simulink model "wamjc7"  (Simulink 8.3)
settings: Solver=ode4  SolverMode=SingleTasking  StartTime=0.0  StopTime=inf  FixedStep=sample_time  RelTol=1e-3
undefined symbols (not defined in the file): arm_home, arm_home_norest, arm_j2mt, arm_m2jp, b, bit, C, CAN_init, enc_per_rev, FT_init, hand_on, MT_init, puck_I_per_Nm, rotFT2Hand, sample_time, Standard, VL1_init, VL2_init
libraries: xpclib x43, simulink x27, xpcutilitieslib x6, dspmathops x1, dspadpt3 x1, dspindex x1, dspbuff3 x1
(part 2 of 5)

== system wamjc7/Get Arm State/Get FT/Get Force Torque/Recieve and Unpack  Forces and Torques ==
  CAN bit-unpacking 1 : xpclib/CAN/Utilities/CAN bit-unpacking   bitpatterns={[0:15],[16:31],[32:47]}  dtypes={'int32','int32','int32'}
  CAN bit-unpacking 2 : xpclib/CAN/Utilities/CAN bit-unpacking   bitpatterns={[0:15],[16:31],[32:47]}  dtypes={'int32','int32','int32'}
  DocBlock : simulink/Model-Wide Utilities/DocBlock  DocumentType=Text
  ForceToDouble : DataTypeConversion  OutDataTypeStr=double
  Mux1 : Mux  Inputs=3
  Mux2 : Mux  Inputs=3
  "Receive position " : xpclib/CAN/Softing/CAN-AC2-PCI SJA 1000/Receive   board=1  canPort=CAN 1  range=Standard (11-bit)  ids=[bin2dec('10100001010'),bin2dec('10100001011')]  lengths=0  output=Data  inten=on  ts=sample_time  ididx=[8,9]
  TorqueToDouble : DataTypeConversion  OutDataTypeStr=double
  F : Outport
  Tau : Outport  Port=2
  wires:
  "Receive position "/1 -> CAN bit-unpacking 2/1
  "Receive position "/2 -> CAN bit-unpacking 1/1
  Mux1/1 -> TorqueToDouble/1
  CAN bit-unpacking 1/1 -> Mux1/1
  CAN bit-unpacking 1/2 -> Mux1/2
  CAN bit-unpacking 1/3 -> Mux1/3
  TorqueToDouble/1 -> Tau/1
  ForceToDouble/1 -> F/1
  CAN bit-unpacking 2/1 -> Mux2/1
  CAN bit-unpacking 2/2 -> Mux2/2
  CAN bit-unpacking 2/3 -> Mux2/3
  Mux2/1 -> ForceToDouble/1

== system wamjc7/Get Arm State/Get FT/Get Force Torque/Send Get FT ==
  Bit Packing : xpcutilitieslib/Bit Packing   MaskBitPatterns={[0:7]}  MaskPackDataType=double  MaskPackDataSize=[1]
  Send to FTsensor : xpclib/CAN/Softing/CAN-AC2-PCI SJA 1000/Send   board=1  canPort=CAN 1  range=Standard (11-bit)  ids=bin2dec('00000001000')  sizes=[1]  output=off  ts=sample_time  ididx=[0]
  get FT : Constant  Value=[54]  OutDataTypeStr=int8
  wires:
  get FT/1 -> Bit Packing/1
  Bit Packing/1 -> Send to FTsensor/1

== system wamjc7/Subsystem/Plan Arm Trajectory/Send Execution Result/Enabled Subsystem ==
  ExectuionResult : Inport
  Enable : EnablePort
  Pack : xpclib/UDP/Pack  datatypes={'double'}  byteAlign=1
  Send : xpclib/UDP/Send  ipAddress=192.168.1.11  ipPort=3334  localPort=-1  vblLen=off  sampletime=sample_time
  wires:
  ExectuionResult/1 -> Pack/1
  Pack/1 -> Send/1

== matlab function Subsystem/Compute Arm Torque/Dynamics Compensation ==
  data: hand_on input double; tau output double; q input double; qd input double; qdd input double; FTsensor output double
function [tau, FTsensor] = dynamicsComp(hand_on,q,qd,qdd)
%-------------------------------------------------------------------------------------
%   SETUP THE ARM
%-------------------------------------------------------------------------------------    
    DH_a = [0 0 0.045 -0.045 0 0 0];
    DH_d = [0 0 .55 0 0.3 0 0.061];
    DH_alpha = [-pi/2 pi/2 -pi/2 pi/2 -pi/2 pi/2 0];

    m = [8.3936 4.8487 1.7251 2.17266212 0.35655692 0.40915886 0.07548270];
    
    com = zeros(3,7);
    com(:,1) = [0.3506e-3, 132.6795e-3, 0.6286e-3];
    com(:,2) = [-0.2230e-3, -21.3924e-3, 13.3754e-3];
    com(:,3) = [-38.7565e-3, 217.9078e-3, 0.0252e-3];
    com(:,4) = [0.00553408,0.00006822,0.11927695];
    com(:,5) = [0.00005483,0.02886286,0.00148493];
    com(:,6) = [-0.00005923,-0.01686123,0.02419052];
    com(:,7) = [ 0.00014836,0.00007252,-0.00335185];
    
    % Need Inertia matricies
    I = zeros(3,3,7);
    I(:,:,1) = [ 95157.4294e-6,   246.1404e-6,   -95.0183e-6 ;
                   246.1404e-6, 92032.3524e-6,  -962.6725e-6 ;
                   -95.0183e-6,  -962.6725e-6, 59290.5997e-6 ];
    I(:,:,2) = [ 29326.8098e-6,   -43.3994e-6,  -129.2942e-6 ;
                   -43.3994e-6, 20781.5826e-6,  1348.6924e-6 ;
                  -129.2942e-6,  1348.6924e-6, 22807.3271e-6 ];
    I(:,:,3) = [ 56662.2970e-6, -2321.6892e-6,     8.2125e-6 ;
                 -2321.6892e-6,  3158.0509e-6,   -16.6307e-6 ;
                     8.2125e-6,   -16.6307e-6, 56806.6024e-6 ];
    I(:,:,4) = [  0.01067491,  0.00004503, -0.00135557 ;
                  0.00004503,  0.01058659, -0.00011002 ;
                 -0.00135557, -0.00011002,  0.00282036 ];
    I(:,:,5) = [  0.00037112, -0.00000008, -0.00000003 ;
                 -0.00000008,  0.00019434, -0.00001613 ;
                 -0.00000003, -0.00001613,  0.00038209 ];
    I(:,:,6) =  [  0.00054889,  0.00000019, -0.00000010 ;
                   0.00000019,  0.00023846, -0.00004430 ;
                  -0.00000010, -0.00004430,  0.00045133 ];
    I(:,:,7) = [ 0.00003911, 0.00000019, 0.00000000 ;      % WAM without hand
                 0.00000019, 0.00003877, 0.00000000 ;
                 0.00000000, 0.00000000, 0.00007614 ];
    
    %Link Gear Ratio
    % The differential drive mechanism was ignored here because it's not
    % supported by the robotic toolbox yet.
    % Please refer to: http://www.me.unm.edu/~starr/research/WAM_MassParams_AA-00.pdf
    G = zeros(7,1);
    G(1) =  42.00;
    G(2) =  28.25;
    G(3) =  28.25;
    G(4) =  18.00;
    G(5) =  9.70;
    G(6) =  9.70;
    G(7) =  14.93;
    %Link Motor Inertia
    Jm = zeros(7,1);
    Jm(1) = 0.00011631;
    Jm(2) = 0.00011831;
    Jm(3) = 0.00011831;
    Jm(4) = 0.00010686;
    Jm(5) = 0.00001685;
    Jm(6) = 0.00001745;
    Jm(7) = 0.00000142;
             
    if hand_on
        hand_mass = 1.3731;
        DH_d(7) = DH_d(7) + .0953; % Adding the distance to the hand frame for the Schunk Gripper
        com(:,7) = ([0.001127;	-0.000211;	0.054851].*hand_mass + com(:,7).*m(7))/(hand_mass + m(7)); % Finding the combined center of mass
        m(7) = m(7) + hand_mass; % Adding the mass of the hand
        I(:,:,7) = [ .003167342,          0,         0;       % Approximate Inertia Tensor for Schunk Gripper
                              0, .001128942,         0;
                              0,          0, .00258007;];
    end
    
%-------------------------------------------------------------------------------------
%  END SETUP OF THE ARM
%-------------------------------------------------------------------------------------

    z0 = [0;0;1];
    grav = [0 0 9.81];
	fext = zeros(6, 1);
    n = 7;
    FTsensor = zeros(6,1);
    
    tau = zeros(n,1);
    
    Fm = zeros(3,7);
    Nm = zeros(3,7);
    N = zeros(3,1);
    pstarm = zeros(3,7);
    Rm = zeros(3,3,7);
    w = zeros(3,1);
    wd = zeros(3,1);
    v = zeros(3,1);
    vd = grav(:);
    
    
    %
	% init some variables, compute the link rotation matrices
	%
    for j=1:n,
        a = DH_a(j);
        d = DH_d(j);
        alpha = DH_alpha(j);
        Tj = getTransformDH(a, d, alpha, q(j));
        
        pstar = [a; d*sin(alpha); d*cos(alpha)];
        if j == 1,
            pstar = eye(3) * pstar;
            Tj = eye(4) * Tj;
        end
        pstarm(:,j) = pstar;
        Rm(:,:,j) = Tj(1:3,1:3);
    end
    
    %
	%  the forward recursion
	%
    for j=1:n,
        Rt = Rm(:,:,j)';	% transpose!!
        pstar = pstarm(:,j);
        r = com(:,j)';

        %
        % statement order is important here
        %
        % revolute axis
        wd = Rt*(wd + z0*qdd(j) + cross(w,z0*qd(j)));
        w = Rt*(w + z0*qd(j));
        %v = cross(w,pstar) + Rt*v;
        vd = cross(wd,pstar) + cross(w, cross(w,pstar)) + Rt*vd;

        %vhat = cross(wd,r') + cross(w,cross(w,r')) + vd;
        vhat = cross(wd,r') + cross(w,cross(w,r')) + vd;
        F = m(j)*vhat;
        N = I(1:3,1:3,j)*wd + cross(w,I(1:3,1:3,j)*w);
        Fm(:,j) = F;
        Nm(:,j) = N;
    end
    
    
    %
	%  the backward recursion
	%

    fext = fext(:);
    f = fext(1:3);		% force/moments on end of arm
    nn = fext(4:6);

    for j=n:-1:1,
        pstar = pstarm(:,j);

        %
        % order of these statements is important, since both
        % nn and f are functions of previous f.
        %
        if j == n,
            R = eye(3,3);
        else
            R = Rm(:,:,j+1);
        end
        r = com(:,j)';
        
        % The expected force/torque at the sensor.  Used for dynamic compensation
        % of the gripper.
        if j == n
            FTsensor(1:3) = R*f + Fm(:,j);
            FTsensor(4:6) = cross(r',Fm(:,j));
        end
        
        nn = R*(nn + cross(R'*pstar,f)) + cross(pstar+r',Fm(:,j)) + Nm(:,j);
        f = R*f + Fm(:,j);
        
        R = Rm(:,:,j);
        % revolute
        tau(j) = nn'*(R'*z0) + G(j)^2 * Jm(j)*qdd(j);% + abs(G(j)) * friction(link, qd(j));
    end

end

function T = getTransformDH(a,d,alpha,q)
    ct = cos(q);
    st = sin(q);
    cb = cos(alpha);
    sb = sin(alpha);
    
    T = [ ct, -st*cb,  st*sb, a*ct;
          st,  ct*cb, -ct*sb, a*st;
          0, sb, cb, d;
          0, 0, 0, 1 ];
end

== matlab function Subsystem/Impedance Controller/Convert NaN to Zero ==
  data: u input double; y output double
function y = fcn(u)
%#eml

u(isnan(u)) = 0; % convert NaN into 0!!!!
u(isinf(u)) = 0;

y = u;

== matlab function Subsystem/Compute Arm Torque/Compute Tool Configuration ==
  data: q input double; w output double; hand_on input double
function w = tool_config(q,hand_on)
    % a, d, and alpha (b) DH parameters
    dh_a = [0 0 0.045 -0.045 0 0 0 0];
    dh_d = [0 0 0.55 0 0.3 0 .061 0]; % Not sure about dh_d(8) For the hand
    dh_b = [-pi/2 pi/2 -pi/2 pi/2 -pi/2 pi/2 0 0];
    
    % hand on
    if (hand_on)
        dh_d(8) = 0.0953; % Schunk Gripper
    end
    
    qFull = [q; 0];
        
    ct = cos(qFull);
    st = sin(qFull);
    cb = cos(dh_b);
    sb = sin(dh_b);

    % compute forward kinematics
    T0 = eye(4);
    for i=1:8
        T = [ ct(i), -st(i)*cb(i),  st(i)*sb(i), dh_a(i)*ct(i);
              st(i),  ct(i)*cb(i), -ct(i)*sb(i), dh_a(i)*st(i);
              0, sb(i), cb(i), dh_d(i);
              0, 0, 0, 1 ];
        T0 = T0*T;
    end

    w = [ T0(1:3,4); T0(1:3,3) ];
end

== matlab function Subsystem/Plan Arm Trajectory/Check FT ==
  data: type input double; guarded input double; FT input double; FTerror output double; InContact output double; FTExp input double; contact_scenario output double; FTERR output double; CTS output double
function [FTerror, InContact,contact_scenario, FTERR,CTS]  = verify_FT(type, guarded, FT, FTExp)
    persistent ErrorCounts type_last ContactCounts AxisBlocked_counts;
    
    % Initialize ErrorCounts
    if isempty(ErrorCounts) || isempty(ContactCounts) || isempty(type_last) || isempty(AxisBlocked_counts)
        ErrorCounts = 0;
        ContactCounts = 0;
        type_last = type;
        reset = 1;
        AxisBlocked_counts = -1;
    else
        reset = 0;
    end
    
    if type_last == 0 && (type == 1 || type == 2)
       reset = 1; 
    end
    
    % Assume no error, set to 1 if we should stop.
    FTerror = 0;
    InContact = 0;
    
    % Compute the error (FT has a gripper force in FT(7) and Gripper width in FT(8))
    GripperForce = FT(7);
    GripperWidth = FT(8);
    AxisBlocked = FT(10);
    FErr = -FTExp(1:3) - FT(1:3);
    TauErr = -FTExp(4:6) - FT(4:6);
    FTERR = [GripperForce;FErr;TauErr];
    
    %
    dt = guarded(3);
    adjustMode = guarded(4);
    squeeze = guarded(5);
    
    signal = FTERR;
    
    [ signal_smoothed ] = smooth(signal, reset);
    
    % Get wether contact exists and the contact scenario
    [contact_or_not] = contact_detection(signal_smoothed);
    [contact_scenario LRBest] = contact_mode_detection(signal_smoothed, GripperWidth);

    if adjustMode == 1 || adjustMode == 2 || adjustMode == 3  % If we are backing up, moving left/right, moving up/down
        contact_or_not = 0; % Disable contact
    end
    
    FTERR = [contact_or_not+contact_scenario*.1;FErr;TauErr];
    
%     % Axis blocked should only occur when the arm is being held stationary
%     if AxisBlocked && type == 0 && dt < .01 && AxisBlocked_counts == -1
%        AxisBlocked_counts = 100;
%     end
%     if AxisBlocked_counts > 0
%        AxisBlocked_counts = AxisBlocked_counts - 1;
%     elseif AxisBlocked_counts == 0
%        AxisBlocked_counts = -1;
%        InContact = 2;
%        contact_scenario = LRBest;
%     end
    

    % guarded(1) - set to 1 for a guarded move, zero for an unguarded move
    % guarded(2) - the first time that the guarded move should be active (can be used for moves that are only guarded after a certain time)
    % guarded(3) - dt, the current time in the guarded move
    if guarded(1) && dt > guarded(2)
        % If we are in a Jacobian cartesian space move or a trajectory move
        if type == 1 || type == 2
            
            % Error if force error in any direction is greater than 10N 
            % Error if torque error in any direction is greater than 2Nm
            if max(abs(FErr)) > 20 ||  max(abs(TauErr)) > 2

               ErrorCounts = ErrorCounts + 1;
               % There have to be a few errors in a row to trip
               if(ErrorCounts >= 150)
                   FTerror = 1;
                   ErrorCounts = 0;
               end
            else
               % No error, so reset the counter
               ErrorCounts = 0;
            end            
        end
        
        if contact_or_not ~= 0
            ContactCounts = ContactCounts + 1;
            % There have to be several contacts in a row to trip
            if ContactCounts >= 150
                InContact = 1;
                ContactCounts = 0;
            end
        else
            ContactCounts = 0;
        end
        
    end
    CTS = [ErrorCounts ContactCounts];
    type_last = type;

end

% This function decides whether contact happened using the force-torque
% sensor and specified threshold. 
% signal_vector should be a time-averaged 7*1 vector [gripperforce, force, torque]
% threshold is a scalar representing the strictness, recommended value
% between [10, 20]
function [ contact ] =  contact_detection(signal_vector)
    threshold = 16;

    Mus = [-0.337634322861447  -0.130386058335315  -0.098594565877126;
            0.273757011075547  -0.016476289250917  -0.072807232006565;
           -0.000208767802535   0.036818865520259   0.046065050271432];
    Pis = [0.157951625363198   0.195300606091319   0.646747768545482];
    Sigma = zeros(3,3,3);
    Sigma(:,:,1) = [0.204764891913026  -0.096565136348113   0.009147745682555;
                   -0.096565136348113   0.238887381134154  -0.038984546927037;
                    0.009147745682555  -0.038984546927037   0.075270646313585];
    Sigma(:,:,2) = [0.099889296660488   0.035874721853541   0.033846034465123;
                    0.035874721853541   0.105346220734475   0.028666422935959;
                    0.033846034465123   0.028666422935959   0.155774067788949];
    Sigma(:,:,3) = [0.054725825465771   0.003368648301894  -0.014556274228691;
                    0.003368648301894   0.044490552114301  -0.004333417130894;
                   -0.014556274228691  -0.004333417130894   0.045027482383305];
    m_nc = [ -0.052387061108295   0.032833282827717  -0.079498518372937  -0.059858140113800   0.002470515976984   0.002255694209123  0.000276539576848];
    pca_vector_nc = [-0.004188538649641   0.027820200838378  -0.014237746479798   0.999495221975548   0.003443678359730   0.000411892412716  -0.001746944908936;
                     -0.427448016586007  -0.024401593759104   0.902721495939015   0.011730377792682  -0.007815172210556  -0.025143914544832  -0.030915384355590;
                      0.798011594955261  -0.477360371170200   0.364479902258289   0.021682258200983   0.041351251599484  -0.016434509962265  -0.002971827007047;
                      0.423236309103029   0.877633894049199   0.223924886795269  -0.019461679311100  -0.003296799307204  -0.007494207961175  -0.006452189269240;
                     -0.035310632068167   0.022396696121380  -0.011263896600617  -0.004310313793208   0.991135832915610  -0.125220033218201  -0.008706152174191;
                     -0.005501687781820   0.003390152482245   0.042126110498095   0.001191043086522   0.090655724693849   0.664386771964729   0.740644292050432;
                      0.006485439767152  -0.001821419394632   0.001322390256420  -0.001680718286583   0.087393189431848   0.736173565237476  -0.671089383211312];
    
    nlogL = negative_log_likelihood(Mus, Sigma, Pis, (signal_vector(:) - m_nc(:))' * pca_vector_nc(:, 1:3));
    contact = double(nlogL >= threshold);
end


% This function calculates the negative log-likelihood and posterior
% responsibility given an observation for a known GMM
function [nlogl, post] = negative_log_likelihood(Mus, Sigmas, pis, X)
    k = size(Mus, 1);
    probs = zeros(1, k);
    for i = 1:k
        probs(i) = single_multivariate_gaussian_distribution(Mus(i, :), Sigmas(:, :, i), X); 
    end
    nlogl = -log(sum(probs .* pis));
    
    post = zeros(1, k);
    for i = 1:k
        post(i) = pis(i)*probs(i)/sum(pis.*probs);
    end
end

% This function calculates a single multi-variate gaussian distribution
% probability
function [prob] = single_multivariate_gaussian_distribution(mu, sigma, x)
    k = length(mu);
    mu = mu(:);
    x = x(:);
    prob = 1/((2*pi)^(k/2)*(det(sigma)^0.5))*exp(-0.5*(x-mu)'/(sigma)*(x-mu));
end

% This function decides which contact mode happened using the force-torque
% sensor, current gripper width, annd pre-computed gaussian kernel among three different cases, left
% fingertip, right fingertip and palm 

% It's not a perfect implementation yet. Because the highest success rate
% on training data is now around 90%. The sigma matrices in the parameter
% set file are optimized based on the training data.

% signal_vector should be a time-averaged 7*1 vector [gripperforce, force, torque]
% contactmode = 1 when left fingertip
% contactmode = 2 when right fingertip
% contactmode = 4 when palm

function [ contactmode, LRBest ] = contact_mode_detection(signal_vector, gripper_width)

    % Parameters from Set8
    sigma1 = [0.011958878344803  -0.034577862520242  -0.040028047727885;
             -0.034577862520242   0.317065652599757   0.211101604469568;
             -0.040028047727885   0.211101604469568   2.244619660879594];
    sigma2 = [0.005148714984431  -0.001939773758019   0.001817410780275;
             -0.001939773758019   0.529389506048068  -0.448411334605652;
              0.001817410780275  -0.448411334605652   3.883697095128499];
    sigma3 = [0.033974727475917  -0.076588901043173  -0.006617010900665;
             -0.076588901043173   1.400901014437577   0.212599907484024;
             -0.006617010900665   0.212599907484024   0.105210315698683];

    kernel1 = mode_kernel_fingertip(signal_vector(2:4), 1, gripper_width);
    kernel2 = mode_kernel_fingertip(signal_vector(2:4), 2, gripper_width);
    kernel4 = mode_kernel_fingertip(signal_vector(2:4), 4, gripper_width);

    data_vector = [signal_vector(5:6); signal_vector(1)];
    density1 = N(sigma1, data_vector, kernel1);
    density2 = N(sigma2, data_vector, kernel2);
    density4 = N(sigma3, data_vector, kernel4);

    contactmode = 0;

    % Find the actual contact mode
    if density1 >= density2 && density1 >= density4
        contactmode = 1;
    end
    if density2 >= density4 && density2 >= density1
        contactmode = 2;
    end
    if density4 >= density1 && density4 >= density2
        contactmode = 4;
    end
    
    % Find the best from left fingertip or right fingertip
    % From experiments a right fingertip contact will be detected when
    % there is a left finger contact and vice versa.
    if density1 >= density2
       LRBest = 2;
    else
       LRBest = 1;
    end
    
end

% Multi-variate Gaussian distribution density function
function  density = N(sigma, x, mu)
    density = 1/(2*pi)^(1.5)/sqrt(det(sigma)) * exp(-0.5 * sum((x-mu)' / sigma .* (x-mu)', 2));
end

% Calculate different gaussian kernels
function [ kernel ] = mode_kernel_fingertip(force, mode, gripper_width)
    offset1 = 0.1763;  % from force-torque origin to fingertip
    offset2 = 0.0953;  % from force-torque origin to palm
    
    switch mode
        case 1
            disvec = [0  gripper_width/2  offset1-offset2];
            gfkernel = force(2);
            torquekernel = cross(disvec, force);
            kernel = [torquekernel(1:2)'; gfkernel];
        case 2
            disvec = [0 -gripper_width/2  offset1-offset2];
            gfkernel = -force(2);
            torquekernel = cross(disvec, force);
            kernel = [torquekernel(1:2)'; gfkernel];
        case 4
            disvec = [0  0  0];
            gfkernel = 0;
            torquekernel = cross(disvec, force);
            kernel = [torquekernel(1:2)'; gfkernel];
    end
end

function  [ newdata ] = smooth(data, reset)
    persistent data_window total_count
    
    time_window_size = 20;
    
    total = zeros(size(data,1),1); % Used to sum up the current values
    
    % Initialize the time window of the data with the specified window size,
    % only the specified value at first call will be effective.
    if isempty(data_window) || reset
        data_window = repmat(data,1,time_window_size);
        total_count = 0;
    end
        
    if total_count < time_window_size
        total_count = total_count + 1;
    end
    
    % Move all of the old data to the front by one slot
    for i = 1:time_window_size-1
       data_window(:,i) = data_window(:,i+1);
    end
    % Put data at the end of the window
    data_window(:,end) = data(:);
    
    for i = time_window_size-total_count+1:time_window_size
       total = total + data_window(:,i);
    end
    
    % Calculate the average of the window
    newdata = total / total_count;

end

== matlab function Subsystem/Plan Arm Trajectory/Compute parameters for next step ==
  data: qdes input double; joint_error input double; FT_error input double; queue_in output double; push output double; traj_done input double; pckt input double; x0 input double; tstart input double; t input double; queue_empty input double; udp input double; udp_rcvd input double; q input double; pop output double; rst output double; pckt_new output double; wam_on input double; x0_new output double; tstart_new output double; wam_flip input double; home input double
function [queue_in,push,pop,rst,pckt_new,x0_new,tstart_new] = fcn(qdes,joint_error, FT_error,traj_done,pckt,x0,tstart,t,queue_empty,udp,udp_rcvd,q,wam_on,wam_flip,home)

    PCKT_LENGTH = 749; % A constant for the number of doubles in a UDP packet
    PCKT_END_ZEROS = PCKT_LENGTH - 8;

    % the input the the queue will always be the UDP packet
    % whether or not we actually push it onto the queue is defined below
    queue_in = udp;
    
    % the wam is on
    if (wam_on)
        % don't reset queue, and push whenever UDP is received
        rst = 0;
        push = udp_rcvd;
        
        % if the wam was just flipped on
        if(wam_flip)
            % feed a static trajectory to move to home position, with a=0.5 and v=0.5
            % set J2 and J4 not resting, causes vibration
            pop = 0;
            x0_new = q;
            pckt_new = [0; home; 0.5*ones(PCKT_END_ZEROS,1)];
            tstart_new = t;
        % else if there was an error
        elseif(joint_error || FT_error)
            rst = 1; % Clear all of the commands
            push = 1;
            pop = 1;
            x0_new = qdes;  % qdes has been checked for joint limits
            pckt_new = [0; qdes; zeros(PCKT_END_ZEROS,1)];
            tstart_new = t;
            queue_in = pckt_new;

        % else if the last step of the trajectory is done
        elseif(traj_done)
            if (queue_empty)
                % trajectory finished but queue is empty, so just hold position for now
                pop = 0;
                x0_new = qdes;
                pckt_new = [0; qdes; zeros(PCKT_END_ZEROS,1)];
                tstart_new = t;
            else
                % grab the next packet in the queue
                % pckt_new unused here, will grab the popped element instead
                pop = 1;
                x0_new = qdes;
                pckt_new = zeros(PCKT_LENGTH,1);
                tstart_new = t;
            end
        % otherwise, we're still in the current trajectory step
        else
            % don't change state
            pop = 0;
            x0_new = x0;
            pckt_new = pckt;
            tstart_new = tstart;
        end
    % the wam is off
    else
        % reset queue, and don't push on anything new
        rst = 1;
        push = 0;
        % set start and desired position to the current position
        pop = 0;
        x0_new = q;
        pckt_new = [0; q; zeros(PCKT_END_ZEROS,1)];
        tstart_new = t;
    end
end
